simulink model "gSSVEP_gMOBIlabplus_8ch"  (Simulink 7.9)
settings: Solver=FixedStepDiscrete  StartTime=0.0  StopTime=260  FixedStep=1/256  RelTol=1e-3
undefined symbols (not defined in the file or in its folder): COM1
libraries: gRTanalyze x2, dspstat3 x2, gMOBIlab x2, dspbuff3 x1, simulink x1, gSTIMboxlib x1
Description:
  | gMOBIlab+ based SSVEP BCI system
  | 
  | Copyright g.tec medical engineering GmbH
settings Model: Creator=g.tec medical engineering GmbH  ModifiedByFormat=g.tec  LastModifiedBy=g.tec
settings DebuggingCC: FcnCallInpInsideContextMsg=Use local settings  StrictBusMsg=Warning
settings GRTTargetCC: CombineOutputUpdateFcns=off  GRTInterface=on

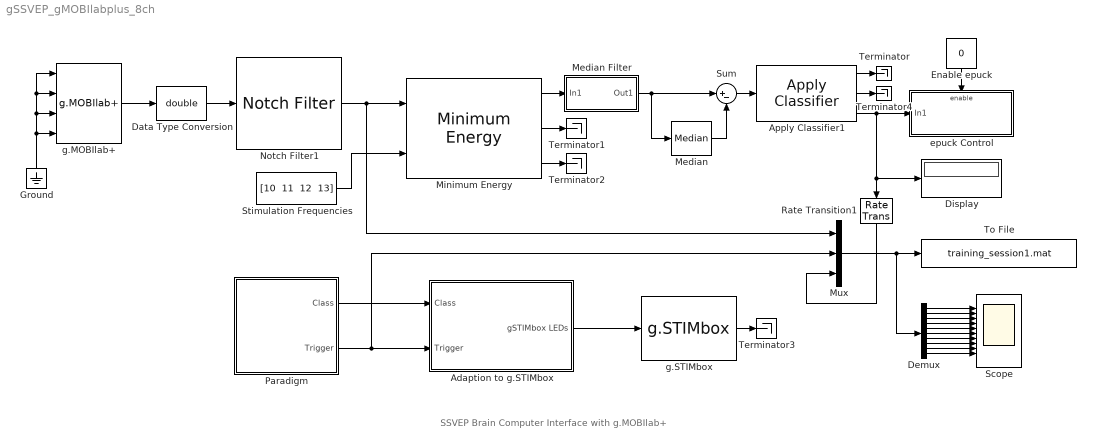
== system gSSVEP_gMOBIlabplus_8ch ==
  note: SSVEP Brain Computer Interface with g.MOBIlab+
  Adaption to g.STIMbox : Subsystem
      settings: MinAlgLoopOccurrences=on
  Apply Classifier1 : gRTanalyze/Apply Classifier
  Data Type Conversion : DataTypeConversion  OutDataTypeStr=double
  Demux : Demux  Outputs=10
  Display : Display
  Enable epuck : Constant  Value=0
  Ground : Ground
  Median : dspstat3/Median  sortAlg=Quick sort  directionMode=Entire input  dimension=1  treatSBRowAsCol=on  outputDataTypeStr=Inherit: Same as accumulator  outputLastDataTypeStr=Inherit: Same as accumulator  outputMin=[]  outputMax=[]  accumDataTypeStr=Inherit: Same as product output  accumLastDataTypeStr=Inherit: Same as product output  roundingMode=Floor  overflowMode=off
      settings: allowOverrides=off
  Median Filter : Subsystem  mask(Moving Median Filter){buflen=10}
      mask prompts: buflen "Filter Length"
      mask help:
      | Smoothes the input channels over time by computing the median value for
      | the specified number of samples.
      mask init:
      | blockhandle = get_param(gcb,'Handle');
      | sysname = get(blockhandle,'Path');
      | syspath = [ sysname '/' ];
      | name = [ syspath get(blockhandle,'Name') ];
      | path = [ name '/' ];
      | if buflen < 3
      |   buflen = 10;
      |   set_param(name,'buflen',num2str(buflen));
      | end
      | set_param([ path 'Collect'],'siz',num2str(buflen));
      | try
      |   set_param([ path 'Collect'],'TreatMby1Signals','M channels (this choice will be removed - see release notes)');
      | catch
      | end
      mask Help:
      | Smoothes the input channels over time by computing the median value for
      | the specified number of samples.
      | 
      | Filter Length ... The length of the smoothing window in samples. (Default 10)
  Minimum Energy : gRTanalyze/Minimum Energy  bufflen=768  reprate=0.20  numharmonics=1  modelorder=7
  Mux : Mux  Inputs=3
  Notch Filter1 : gMOBIlab/Notch Filter  notch=50Hz
  Paradigm : Subsystem  mask{classinfo=classinfo_20tr.m, mode=Training Paradigm, trialperiod=10.5, activepart=70, initialoffset=10}
      mask prompts: classinfo "Class Info File"; trialperiod "Trial Period [s] (>= 8s)"; activepart "Active Part [%]"; initialoffset "Initial Offset [s] (>= 10s)"
      mask init:
      | blockhandle = get_param(gcb,'Handle');
      | sysname = get(blockhandle,'Path');
      | syspath = [ sysname '/' ];
      | name = [ syspath get(blockhandle,'Name') ];
      | path = [ name '/' ];
      | rootsys = bdroot(name);
      | 
      | if ~strcmp(get_param(rootsys, 'SolverType'),'Fixed-step')
      |         set_param(rootsys, 'SolverType','Fixed-step');
      | end
      |         
      | stepsize = get_param(rootsys,'FixedStep');
      | if strcmp(stepsize,'auto')
      |     error('Currently not known how to determine FixedStep size during initialization')
      | end
      | 
      | if mode==3    %Free Running
      |     paradigmDrivePattern = [ 0 , -1 ];
      |     
      | else   %Training paradigm or Paradigm with feedback
      |     try 
      |       ci = load(classinfo);
      |       [ cival ci ] = max(ci',[],1);
      |      % ci(end +1) = 0;
      |     catch
      |       fprintf(2,'File %s required check paths and session settings\n', classinfo);
      |       error('File %s required check paths and session settings', classinfo);
      |     end
      |  %   set_param([ path 'SetTrigger' ],'Value','1');
      |     
      |     if trialperiod < 8   %trialperiod should not be higher than 5s (could be removed if necessary)
      |       trialperiod = 8;
      |       set_param(name,'trialperiod','5');
      |     end
      |     if activepart > 95   %activepart should be lower than 95% (could be removed if necessary)
      |       activepart = 95;
      |       set_param(name,'activepart','95');
      |     end
      |     if initialoffset < 10   %initaloffset should be >= 0s
      |       initialoffset = 10;
      |       set_param(name,'initialoffset','0');
      |     end
      |     
      |     hightime = activepart / 100 * trialperiod;
      | 
      |     stepsize_int = str2num(stepsize);
      |     hightime = round(hightime / stepsize_int);
      |     trialperiod = round(trialperiod / stepsize_int);
      |     if hightime < 2 / stepsize_int    %hightime should not be lower than 2s (could be removed if necessary)
      |         hightime = 2 / stepsize_int;
      |     end
      |         
      |     offset_samp = round(initialoffset / stepsize_int);
      |         
      |     %activepart = hightime;
      |     array = zeros(1,trialperiod*size(ci,2)+offset_samp);
      |     for cnt=1:size(ci,2)
      |         put = ( cnt - 1) * trialperiod + 1 + offset_samp;
      |         put = put:(put+hightime-1);
      |         array(1,put) = ci(cnt);
      |     end
      |     ci=array;
      |     ci = [ [0:( size(ci,2) - 1 )].*stepsize_int ; ci ];
      |     paradigmDrivePattern = ci';
      |             
      |     period = num2str(trialperiod,10);
      |     offset = num2str(initialoffset,10);
      | end
      | 
      | set_param([ path 'Class Info' ],'VariableName','paradigmDrivePattern');
      | set_param([ path 'Class Info' ],'SampleTime',stepsize);
      | 
      | clear blockhandle sysname syspath name path classinfo trialperiod activepart initialoffset
      settings: MinAlgLoopOccurrences=on
      mask StyleString: edit,popup(Training Paradigm|Paradigm with feedback|Free running),edit,edit,edit
  Rate Transition1 : RateTransition
  Scope : Scope  NumInputPorts=10
      settings: TickLabels=off  TimeRange=15  YMin=-50~-50~-50~-50~-50~-50~-50~-50~-1~0  YMax=50~50~50~50~50~50~50~50~2~5
  Stimulation Frequencies : Constant  Value="[10  11  12  13]"  SampleTime=1/256
  Sum : Sum  Inputs=|+-
  Terminator{,1..4} (5 alike) : Terminator
  To File : ToFile  Filename=training_session1.mat  MatrixName=y
  epuck Control : Subsystem  TreatAsAtomicUnit=on  mask{com='com30'}
      mask prompts: com "Com - Port (COMxx)"
  g.MOBIlab+ : gMOBIlab/g.MOBIlab+  analog_channel1=on  analog_channel2=on  analog_channel3=on  analog_channel4=on  analog_channel5=on  analog_channel6=on  analog_channel7=on  analog_channel8=on  dio1=OFF  dio2=OFF  dio3=OFF  dio4=OFF  dio5=OFF  dio6=OFF  dio7=OFF  dio8=OFF  max_delay=10000  port=COM1:  SDflag=off  filename='GMOBILAB'  testmode=off  NoCh1=50 Hz  NoCh2=50 Hz  NoCh3=50 Hz  NoCh4=50 Hz  NoCh5=50 Hz  NoCh6=50 Hz  NoCh7=50 Hz  NoCh8=50 Hz
  g.STIMbox : gSTIMboxlib/g.STIMbox  comport=18  sr=32  fl=1  ia=1  bm=0  fs=1  chmodes="[0  0  0  0  0  0  0  0  1  0  1  0  1  0  1  0]"  chfreqs="[1   1   1   1   1   1   1   1  10   1  11   1  12   1  13   1]"  chinv="[0  0  0  0  0  0  0  0  0  0  0  0  0  0]"
  wires:
  Apply Classifier1/3 -> Rate Transition1/1, Display/1, epuck Control/1(In1)
  Stimulation Frequencies/1 -> Minimum Energy/2
  Minimum Energy/1 -> Median Filter/1(In1)
  Median Filter/1(Out1) -> Sum/1, Median/1
  Minimum Energy/2 -> Terminator1/1
  Minimum Energy/3 -> Terminator2/1
  Notch Filter1/1 -> Mux/1, Minimum Energy/1
  Paradigm/2(Trigger) -> Mux/2, Adaption to g.STIMbox/2(Trigger)
  Mux/1 -> To File/1, Demux/1
  Paradigm/1(Class) -> Adaption to g.STIMbox/1(Class)
  Rate Transition1/1 -> Mux/3
  Adaption to g.STIMbox/1(gSTIMbox LEDs) -> g.STIMbox/1
  Enable epuck/1 -> epuck Control/Enable
  g.STIMbox/1 -> Terminator3/1
  Demux/1 -> Scope/1
  Demux/2 -> Scope/2
  Demux/3 -> Scope/3
  Demux/4 -> Scope/4
  Demux/5 -> Scope/5
  Demux/6 -> Scope/6
  Demux/7 -> Scope/7
  Demux/8 -> Scope/8
  Demux/9 -> Scope/9
  Demux/10 -> Scope/10
  g.MOBIlab+/1 -> Data Type Conversion/1
  Data Type Conversion/1 -> Notch Filter1/1
  Ground/1 -> g.MOBIlab+/1, g.MOBIlab+/2, g.MOBIlab+/3, g.MOBIlab+/4
  Median/1 -> Sum/2
  Sum/1 -> Apply Classifier1/1
  Apply Classifier1/1 -> Terminator/1
  Apply Classifier1/2 -> Terminator4/1

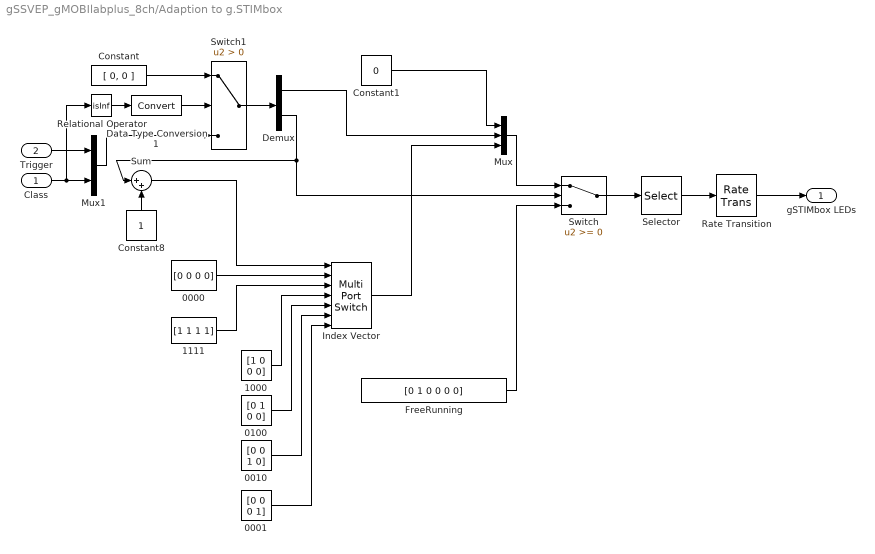
== system gSSVEP_gMOBIlabplus_8ch/Adaption to g.STIMbox ==
  Class : Inport
  Trigger : Inport  Port=2
  0000 : Constant  Value=[0 0 0 0]  SampleTime=1/256
  0001 : Constant  Value=[0 0 0 1]  SampleTime=1/256
  0010 : Constant  Value=[0 0 1 0]  SampleTime=1/256
  0100 : Constant  Value=[0 1 0 0]  SampleTime=1/256
  1000 : Constant  Value=[1 0 0 0]  SampleTime=1/256
  1111 : Constant  Value=[1 1 1 1]  SampleTime=1/256
  Constant : Constant  Value=[ 0, 0 ]
  Constant1 : Constant  Value=0  SampleTime=1/256
  Constant8 : Constant  SampleTime=1/256
  Data Type Conversion1 : DataTypeConversion
  Demux : Demux  Outputs=2
  FreeRunning : Constant  Value=[0 1 0 0 0 0]  SampleTime=1/256
  Index Vector : MultiPortSwitch  DataPortOrder=Zero-based contiguous  Inputs=6  zeroidx=on
  Mux : Mux  Inputs=3
  Mux1 : Mux  Inputs=2
  Rate Transition : RateTransition
  Relational Operator : RelationalOperator  Operator=isInf  OutDataTypeStr=boolean
  Selector : Selector  InputPortWidth=6  IndexOptions=Index vector (dialog)  Indices=[ones(1,8) 2 3 2 4 2 5 2 6]  OutputSizes=1
  Sum : Sum  Inputs=|++
  Switch : Switch
  Switch1 : Switch  Criteria=u2 > Threshold
  gSTIMbox LEDs : Outport
  wires:
  Trigger/1 -> Mux1/1
  Constant1/1 -> Mux/1
  Index Vector/1 -> Mux/3
  Mux/1 -> Switch/1
  FreeRunning/1 -> Switch/3
  Switch/1 -> Selector/1
  Selector/1 -> Rate Transition/1
  Rate Transition/1 -> gSTIMbox LEDs/1
  Class/1 -> Relational Operator/1, Mux1/2
  Constant8/1 -> Sum/2
  Sum/1 -> Index Vector/1
  0000/1 -> Index Vector/2
  1111/1 -> Index Vector/3
  1000/1 -> Index Vector/4
  0100/1 -> Index Vector/5
  0010/1 -> Index Vector/6
  0001/1 -> Index Vector/7
  Relational Operator/1 -> Data Type Conversion1/1
  Data Type Conversion1/1 -> Switch1/2
  Constant/1 -> Switch1/1
  Switch1/1 -> Demux/1
  Mux1/1 -> Switch1/3
  Demux/1 -> Mux/2
  Demux/2 -> Sum/1, Switch/2

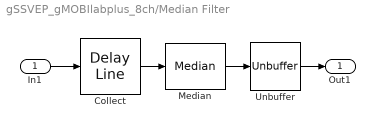
== system gSSVEP_gMOBIlabplus_8ch/Median Filter ==
  In1 : Inport
  Collect : dspbuff3/Delay Line  siz=10  ic=0  directfeed=on  enable_output=off  hold_output=off  TreatMby1Signals=M channels (this choice will be removed - see release notes)
  Median : dspstat3/Median  sortAlg=Quick sort  directionMode=Specified dimension  dimension=1  treatSBRowAsCol=on  outputDataTypeStr=Inherit: Same as accumulator  outputLastDataTypeStr=Inherit: Same as accumulator  outputMin=[]  outputMax=[]  accumDataTypeStr=Inherit: Same as product output  accumLastDataTypeStr=Inherit: Same as product output  roundingMode=Floor  overflowMode=off
      settings: allowOverrides=off
  Unbuffer : Unbuffer
  Out1 : Outport
  wires:
  Unbuffer/1 -> Out1/1
  Median/1 -> Unbuffer/1
  Collect/1 -> Median/1
  In1/1 -> Collect/1

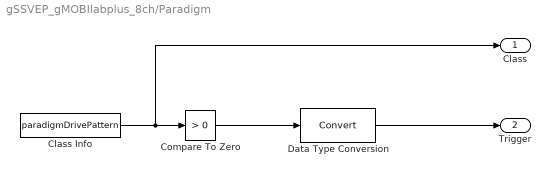
== system gSSVEP_gMOBIlabplus_8ch/Paradigm ==
  Class Info : FromWorkspace  VariableName=paradigmDrivePattern  SampleTime=1/256  Interpolate=off  OutputAfterFinalValue=Holding final value
  Compare To Zero : simulink/Logic and Bit Operations/Compare To Zero  relop=>  OutDataTypeStr=uint8  ZeroCross=off
  Data Type Conversion : DataTypeConversion
  Class : Outport  InitialOutput=0
  Trigger : Outport  Port=2  InitialOutput=0
  wires:
  Class Info/1 -> Compare To Zero/1, Class/1
  Compare To Zero/1 -> Data Type Conversion/1
  Data Type Conversion/1 -> Trigger/1

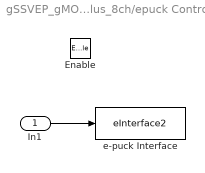
== system gSSVEP_gMOBIlabplus_8ch/epuck Control ==
  In1 : Inport
  Enable : EnablePort  PropagateVarSize=During execution
  e-puck Interface : M-S-Function  FunctionName=eInterface2  Parameters=f b l r s com vmax vmin a  mask(Paramteters ){f=2, b=4, l=1, r=3, s=0, vmax=300, vmin=50, a=1}
      mask prompts: f "Forward"; b "Backward"; l "Left"; r "Right"; s "Stop"; vmax "max. Speed"; vmin "min. Speed"; a "Acceleration"
      mask help:
      | Speed from 0 to 1000;
      | If Acceleration [cm/s] equal 0, then speed of robot = vmin;
      | Forward, Backward, Left, Right and Stop have to have different numbers;
      mask Display: port_label('input', 1, 'Command')
  wires:
  In1/1 -> e-puck Interface/1
